simulink model "D53_LKAS_JLU_20200903_0931"  (R2018b)
settings: Solver=ode3  StartTime=0.0  StopTime=10.0  FixedStep=0.01  RelTol=1e-3  EnableMultiTasking=on
model workspace (MAT data in the model file):
  MCOS : class17 (value not decoded)
  MCOS : class17 (value not decoded)
  MCOS : class17 (value not decoded)
  MCOS : class17 (value not decoded)
  MCOS : class17 (value not decoded)
  MCOS : class17 (value not decoded)
  MCOS : class17 (value not decoded)
  MCOS : class17 (value not decoded)
  MCOS : class17 (value not decoded)
  MCOS : class17 (value not decoded)
  MCOS : class17 (value not decoded)
  MCOS : class17 (value not decoded)
  MCOS : class17 (value not decoded)
  MCOS : class17 (value not decoded)
  MCOS : class17 (value not decoded)
  MCOS : class17 (value not decoded)
  MCOS : class17 (value not decoded)
  MCOS : class17 (value not decoded)
  MCOS : class17 (value not decoded)
  MCOS : class17 (value not decoded)
  MCOS : class17 (value not decoded)
  MCOS : class17 (value not decoded)
  MCOS : class17 (value not decoded)
  MCOS : class17 (value not decoded)
  MCOS : class17 (value not decoded)
  MCOS : class17 (value not decoded)
  MCOS : class17 (value not decoded)
  MCOS : class17 (value not decoded)
  MCOS : class17 (value not decoded)
  MCOS : class17 (value not decoded)
  MCOS : class17 (value not decoded)
  MCOS : class17 (value not decoded)
  MCOS : class17 (value not decoded)
  MCOS : class17 (value not decoded)
  MCOS : class17 (value not decoded)
  MCOS : class17 (value not decoded)
  MCOS : class17 (value not decoded)
  MCOS : class17 (value not decoded)
  MCOS : class17 (value not decoded)
  MCOS : class17 (value not decoded)
  MCOS : class17 (value not decoded)
  MCOS : class17 (value not decoded)
  MCOS : class17 (value not decoded)
  MCOS : class17 (value not decoded)
  MCOS : class17 (value not decoded)
  MCOS : class17 (value not decoded)
  MCOS : class17 (value not decoded)
  MCOS : class17 (value not decoded)
  MCOS : class17 (value not decoded)
  MCOS : class17 (value not decoded)
  MCOS : class17 (value not decoded)
  MCOS : class17 (value not decoded)
  MCOS : class17 (value not decoded)
  MCOS : class17 (value not decoded)
  MCOS : class17 (value not decoded)
  MCOS : class17 (value not decoded)
  MCOS : class17 (value not decoded)
  MCOS : class17 (value not decoded)
  MCOS : class17 (value not decoded)
  MCOS : class17 (value not decoded)
  MCOS : class17 (value not decoded)
  MCOS : class17 (value not decoded)
  MCOS : class17 (value not decoded)
  MCOS : class17 (value not decoded)
  MCOS : class17 (value not decoded)
  MCOS : class17 (value not decoded)
  MCOS : class17 (value not decoded)
  MCOS : class17 (value not decoded)
  MCOS : class17 (value not decoded)
  MCOS : class17 (value not decoded)
  MCOS : class17 (value not decoded)
  MCOS : class17 (value not decoded)
  MCOS : class17 (value not decoded)
  MCOS : class17 (value not decoded)
  MCOS : class17 (value not decoded)
  MCOS : class17 (value not decoded)
  MCOS : class17 (value not decoded)
  MCOS : class17 (value not decoded)
  MCOS : class17 (value not decoded)
  MCOS : class17 (value not decoded)
  MCOS : class17 (value not decoded)
  MCOS : class17 (value not decoded)
  MCOS : class17 (value not decoded)
  MCOS : class17 (value not decoded)
  MCOS : class17 (value not decoded)
  MCOS : class17 (value not decoded)
  MCOS : class17 (value not decoded)
  MCOS : class17 (value not decoded)
  MCOS : class17 (value not decoded)
undefined symbols (not defined in the file): LKA_CarWidth, LKA_SampleTime, LKA_StrRatio_C, LKA_Veh2CamL_C, LKA_Veh2CamW_C, LKA_WhlBaseL_C, LL_CompSWA_C, LL_CrvtPrvwT_C, LL_DesDvt_C, LL_DvtComp_C, LL_DvtPrvwT_C, LL_DvtSpdDet_vDvtSpdMin_C, LL_HdAgExT_C, LL_HdAgPrvwT_C, LL_LAccMax_C, LL_LAccRMax_C, LL_LDW_EarliestWarnLine_C, LL_LDW_LatestWarnLine_C, LL_LDWS_SUPPRESS_HEADING, LL_LFClb_TFC_DiffCtlBalance, LL_LFClb_TFC_DiffCtrlMaxSWA, LL_LFClb_TFC_DiffCtrlRatio, LL_LFClb_TFC_facmGainLutGain1_C, LL_LFClb_TFC_facmGainLutGain2_C, LL_LFClb_TFC_facmIntegRatio, LL_LFClb_TFC_facmKlat_C, LL_LFClb_TFC_FfCtlRatio_C, LL_LFClb_TFC_phiIntegCtlMaxSWA_C, LL_LFClb_TFC_tiKlatPrvwT_C, LL_LFClb_TFC_vGainLutVehSpdLwr_C, LL_LFClb_TFC_vGainLutVehSpdUpr_C, LL_LKA_EarliestWarnLine_C, LL_LKA_LatestWarnLine_C, LL_LKAExPrcs_ExitC0Dvt, LL_LKAExPrcs_ExitC0Swt, LL_LKAExPrcs_tiExitTime1, LL_LKAExPrcs_tiExitTime2, LL_LKAExPrcs_tiExitTime3, LL_LKAS_OUT_OF_CONTROL_LAT_VEL, LL_LKAS_OUT_OF_CONTROL_TTLC, LL_LKASWASyn_M0, LL_LKASWASyn_M1, LL_LKASWASyn_M2, LL_LKASWASyn_M3K, LL_LKASWASyn_SWAaddMax, LL_LKASWASyn_T2, LL_LKASWASyn_tiTrqSwaRtTime, LL_LKASWASyn_tiTrqSwaTime, LL_LKASWASyn_TrqMax, LL_LKASWASyn_TrqSwaAddSwt, LL_LKASWASyn_TrqSwaRateDiff, LL_LSpdCompT_C, LL_lStpLngth_C, LL_MAX_DELAY_EPSSTAR_TIME, LL_MAX_DRIVER_TORQUE_DISABLE, LL_MAX_DRIVER_TORQUE_ENABLE, LL_MAX_LANE_WIDTH_DISABLE, LL_MAX_LANE_WIDTH_ENABLE, LL_MAX_LAT_ACC_DISABLE, LL_MAX_LAT_ACC_ENABLE ... (+30)
libraries: simulink x135, canmsglib x41, dspstat3 x3, simulink_extras x1
(part 8 of 18)

== system D53_LKAS_JLU_20200903_0931/LL/LLOn/LKA/LKA Motion Planning (LKAMP)  ==
  LKAMP_bsInInfoSyn : Inport
  LKAMP_stLKAActvFlg : Inport  Port=2
  LKAMP_bsLKAInPInfo : Inport  Port=3
  LKAMP_bsLKAClb : Inport  Port=4
  LLClb_bsConstantClb : Inport  Port=5
  Add : Sum  OutDataTypeStr=uint8
  Bus Selector : BusSelector  OutputSignals=MPInP_vVehSpdIni
  Bus Selector1 : BusSelector  OutputSignals=bsVehMovInfo.ESC_VehSpd
  Bus Selector2 : BusSelector  OutputSignals=LKA_CarWidth
  Bus Selector3 : BusSelector  OutputSignals=LL_HdAgExT_C,LL_LSpdCompT_C
  Bus Selector4 : BusSelector  OutputSignals=bsVehMovInfo.ESC_VehSpd
  Bus Selector5 : BusSelector  OutputSignals=LW_LaneWidth
  Constant : Constant  OutDataTypeStr=uint8  SampleTime=-1
  Constant19 : Constant  OutDataTypeStr=uint8  SampleTime=-1
  If : If  NumInputs=2  IfExpression=u1==u2  ShowElse=off
  LKA Motion Planning Calculation (LKAMPCal) : Subsystem  Description=|
      | Block Name: LKA Motion Planning Calculation
      | Ab.: LKAMPCal
      | No.: 1.2.3.2
      | Rev: 0.0.1
      | Update Date: 19-3-26
      settings: RTWSystemCode=Nonreusable function
  Memory1 : Memory  InheritSampleTime=on
  Motion Planning Input Processing (MPInP) : Subsystem  Description=|
      | Block Name: Motion Planning Input Processing
      | Ab.: MPInP
      | No.: 1.2.3.1
      | Rev: 0.0.1
      | Update Date: 19-3-26
  Nominal Time Calculation (NomTCalc) : Subsystem  Description=|
      | Block Name: Nominal Time Calculation
      | Ab.: NomTCalc
      | No.: 1.2.3.3
      | Rev: 0.0.1
      | Update Date: 19-3-26
  Saturation1 : Saturate  UpperLimit=5  LowerLimit=0  OutDataTypeStr=uint8
  Saturation6 : Saturate  UpperLimit=2  LowerLimit=0.2
  Steering Wheel Angle Command Calculation (SWACmdCal) : Subsystem  Description=|
      | Block Name: Steering Wheel Angle Command Calculation
      | Ab.: SWACmdCal
      | No.: 1.2.3.4
      | Rev: 0.0.1
      | Update Date: 19-3-26
  Switching Condition (SwtCon) : Subsystem
  LKAMP_phiSWACmd : Outport
  LKAMP_tiT1 : Outport  Port=2
  LKAMP_tiT2 : Outport  Port=3
  wires:
  Bus Selector5/1 -> Switching Condition (SwtCon)/4(SwtCon_lLaneWidth_C)  "<LW_LaneWidth>"
  Saturation6/1 -> LKAMP_tiT1/1
  LKAMP_bsInInfoSyn/1 -> Bus Selector4/1, Bus Selector1/1, Motion Planning Input Processing (MPInP)/4(MPInP_bsInInfoSyn)
  Bus Selector3/2 -> Switching Condition (SwtCon)/7(SwtCon_tiLSpdCompT_C)  "<LL_LSpdCompT_C>"
  LLClb_bsConstantClb/1 -> Bus Selector2/1, LKA Motion Planning Calculation (LKAMPCal)/3(LLClb_bsConstantClb)
  LKAMP_bsLKAInPInfo/1 -> Motion Planning Input Processing (MPInP)/3(MPInP_bsLKAInPInfo), Switching Condition (SwtCon)/2(SwtCon_bsLKAInPInfo), Bus Selector5/1
  Bus Selector2/1 -> Switching Condition (SwtCon)/5(SwtCon_lCarWidth_C)  "<LKA_CarWidth>"
  LKAMP_bsLKAClb/1 -> LKA Motion Planning Calculation (LKAMPCal)/2(LKAMPCal_bsLKAClb), Bus Selector3/1
  LKAMP_stLKAActvFlg/1 -> Motion Planning Input Processing (MPInP)/1(MPInP_stLKAActvFlg), Switching Condition (SwtCon)/1(SwtCon_stLKAActvFlg)
  Bus Selector4/1 -> Switching Condition (SwtCon)/3(SwtCon_vVehSpd)  "<ESC_VehSpd>"
  Bus Selector3/1 -> Switching Condition (SwtCon)/6(SwtCon_tiHdAgExTime_C)  "<LL_HdAgExT_C>"
  Saturation1/1 -> If/1, Memory1/1
  Add/1 -> Saturation1/1
  Constant19/1 -> If/2
  Constant/1 -> Add/1
  Memory1/1 -> Add/2
  If/1 -> LKA Motion Planning Calculation (LKAMPCal)/Action
  LKA Motion Planning Calculation (LKAMPCal)/1(LKAMPCal_bsLKAMPCalOut) -> Steering Wheel Angle Command Calculation (SWACmdCal)/1(SWACmdCal_bsK1K2DetOut)
  Switching Condition (SwtCon)/1(SwtCon_phiHdAgMax) -> Motion Planning Input Processing (MPInP)/2(MPInP_phiHdAgMax)
  Nominal Time Calculation (NomTCalc)/1(NomTCalc_tiNomT) -> Steering Wheel Angle Command Calculation (SWACmdCal)/3(SWACmdCal_tiNomT)
  Bus Selector1/1 -> Nominal Time Calculation (NomTCalc)/1(NomTCalc_vVehSpd)  "<ESC_VehSpd>"
  Bus Selector/1 -> Nominal Time Calculation (NomTCalc)/2(NomTCalc_vVehSpdIni)  "<MPInP_vVehSpdIni>"
  Steering Wheel Angle Command Calculation (SWACmdCal)/1(SWACmdCal_phiSWACmd) -> LKAMP_phiSWACmd/1
  Steering Wheel Angle Command Calculation (SWACmdCal)/2(SWACmdCal_tiT1) -> Saturation6/1
  Motion Planning Input Processing (MPInP)/1(MPInP_bsMPInPInfo) -> LKA Motion Planning Calculation (LKAMPCal)/1(LKAMPCal_bsLKAInPInfo), Bus Selector/1, Steering Wheel Angle Command Calculation (SWACmdCal)/2(SWACmdCal_bsLKAInPInfo)  "LKAMP_bsMPInPInfo"
  Steering Wheel Angle Command Calculation (SWACmdCal)/3(SWACmdCal_tiT2) -> LKAMP_tiT2/1

== system D53_LKAS_JLU_20200903_0931/LL/LLOn/LKA/LKA SWA Limit (LKASWALim) ==
  LKASWALim_phiTFCSWACmd : Inport
  LKASWALim_Ff : Inport  Port=2
  LKASWALim_bsLKAInPInfo : Inport  Port=3
  LKASWALim_bsLKAClb : Inport  Port=4
  Add : Sum  Inputs=+-+  OutDataTypeStr=single
  Add1 : Sum
  Add2 : Sum
  Bus Selector1 : BusSelector  OutputSignals=LKAInP_phiSWAPos,UndrLim_phiSWAMax,UndrLim_dphiSWARMax
  Bus Selector3 : BusSelector  OutputSignals=LL_CompSWA_C
  Gain1 : Gain  Gain=-1.4  OutDataTypeStr=single
  Gain2 : Gain  Gain=-1  OutDataTypeStr=single
  Gain3 : Gain  Gain=1.4  OutDataTypeStr=single
  "Rate Limiter Dynamic " : Subsystem
  Saturation Dynamic : simulink/Discontinuities/Saturation Dynamic  OutMin=[]  OutMax=[]  OutDataTypeStr=Inherit: Same as second input  OutDataType=fixdt(1, 16)  OutScaling=2^-10  DoSatur=off
  LKASWALim_phiSWACmd : Outport
  wires:
  Add2/1 -> Saturation Dynamic/3
  Add1/1 -> Saturation Dynamic/1
  LKASWALim_Ff/1 -> Add1/1, Add2/1
  Bus Selector1/1 -> Add/3  "<LKAInP_phiSWAPos>"
  LKASWALim_bsLKAInPInfo/1 -> Bus Selector1/1
  Add/1 -> Saturation Dynamic/2
  Gain1/1 -> "Rate Limiter Dynamic "/3(lo)
  Gain2/1 -> Add2/2
  Bus Selector1/3 -> Gain1/1, Gain3/1  "<UndrLim_dphiSWARMax>"
  Bus Selector1/2 -> Gain2/1, Add1/2  "<UndrLim_phiSWAMax>"
  LKASWALim_bsLKAClb/1 -> Bus Selector3/1
  LKASWALim_phiTFCSWACmd/1 -> Add/1
  Bus Selector3/1 -> Add/2  "<LL_CompSWA_C>"
  "Rate Limiter Dynamic "/1(Y) -> LKASWALim_phiSWACmd/1
  Saturation Dynamic/1 -> "Rate Limiter Dynamic "/2(u)
  Gain3/1 -> "Rate Limiter Dynamic "/1(up)

== system D53_LKAS_JLU_20200903_0931/LL/LLOn/LKA/Lane Following (LF) ==
  LF_bsInInfoSyn : Inport
  LF_bsLKAInPInfo : Inport  Port=2
  LF_bsLFClb : Inport  Port=3
  LF_bsConstantClb : Inport  Port=4
  Bus Selector4 : BusSelector  OutputSignals=LL_TFCClb
  Preview Information Calculation (PIC) : Subsystem  Description=|
      | Block Name:Preview Information Calculation
      | Ab.: PIC
      | No.: 02.01
      | Rev: 00.00.01
      | Update Date: 19-3-28
  Trajectory Following Control (TFC) : Subsystem  Description=|
      | Block Name:Trajectory Following Control
      | Ab.: TFC
      | No.: 02.02
      | Rev: 00.00.01
      | Update Date: 19-3-28
  LF_phiFfLFSWACmd : Outport
  LF_phiPropSWACmd : Outport  Port=2
  LF_phiIntegSWACmd : Outport  Port=3
  LF_phiDiffSWACmd : Outport  Port=4
  wires:
  LF_bsLKAInPInfo/1 -> Preview Information Calculation (PIC)/1(PIC_bsLKAInPInfo)
  Trajectory Following Control (TFC)/1(TFC_phiFfSWACmd) -> LF_phiFfLFSWACmd/1
  LF_bsInInfoSyn/1 -> Trajectory Following Control (TFC)/2(TFC_bsInInfoSyn)
  Preview Information Calculation (PIC)/1(PIC_bsPrvwInfo) -> Trajectory Following Control (TFC)/1(TFC_bsPrvwInfo)
  Bus Selector4/1 -> Trajectory Following Control (TFC)/3(TFC_bsTFCClb)  "<LL_TFCClb>"
  LF_bsLFClb/1 -> Bus Selector4/1
  LF_bsConstantClb/1 -> Trajectory Following Control (TFC)/4(TFC_bsConstantClb)
  Trajectory Following Control (TFC)/2(TFC_phiPropSWACmd) -> LF_phiPropSWACmd/1
  Trajectory Following Control (TFC)/3(TFC_phiIntegSWACmd) -> LF_phiIntegSWACmd/1
  Trajectory Following Control (TFC)/4(TFC_phiDiffSWACmd) -> LF_phiDiffSWACmd/1

== system D53_LKAS_JLU_20200903_0931/LL/LLOn/LKA/Plan To LaneFollowing (PTLF) ==
  InP : Inport
  Plan : Inport  Port=2
  T1 : Inport  Port=3
  DrvTrq : Inport  Port=4
  Ff : Inport  Port=5
  P : Inport  Port=6
  I : Inport  Port=7
  D : Inport  Port=8
  Add1 : Sum  Inputs=+-
  Add2 : Sum  Inputs=+-
  Add3 : Sum
  Add4 : Sum  Inputs=+++++
  Add5 : Sum  Inputs=+-
  Bus Selector1 : BusSelector  OutputSignals=Pr_bsPrInfo.bsPrCrvtInfo.crPrvwCrvt
  Bus Selector2 : BusSelector  OutputSignals=Pr_bsPrInfo.bsPrHdAgInfo.phiHdAgLft,Pr_bsPrInfo.bsPrHdAgInfo.phiHdAgRgt
  Constant1 : Constant  Value=0.1  OutDataTypeStr=single
  Constant2 : Constant  OutDataTypeStr=single
  Divide : Product  Inputs=*/
  Divide{1..2,5..7} (5 alike) : Product  Inputs=**
  Divide3 : Product  Inputs=*/
  Divide4 : Product  Inputs=*/
  InsideJudge : Subsystem
  InsideJudge1 : Subsystem
  LowPass : Subsystem
  Saturation : Saturate  UpperLimit=1  LowerLimit=0
  Saturation1 : Saturate  UpperLimit=1  LowerLimit=0
  Saturation2 : Saturate  UpperLimit=1  LowerLimit=0
  Saturation3 : Saturate  UpperLimit=0.004  LowerLimit=-0.004
  Saturation6 : Saturate  LowerLimit=0.2
  Switch : Switch  Criteria=u2 > Threshold
  TickTime (TTime) : Subsystem
      mask Display:
      | port_label('output', 1, 'TTime');
      | color('blue');
      | text(0.98,0.9,'VCDC Block','horizontalAlignment','right');
      | color('black');
      | text(0.5,0.55,'Tick Time','horizontalAlignment','center');
      | text(0.5,0.4,'(TTime)','horizontalAlignment','center');
  TimeGain : Subsystem
  SWACmd : Outport
  wires:
  InsideJudge1/2(Plan_1) -> [Plan]
  [Time] -> InsideJudge1/6(Time)
  Plan/1 -> InsideJudge1/5(Plan)
  T1/1 -> InsideJudge1/4(T1)
  Bus Selector2/2 -> InsideJudge1/3(HdAgRgt)  "<phiHdAgRgt>"
  Bus Selector2/1 -> InsideJudge1/2(HdAgLft)  "<phiHdAgLft>"
  [ActFlg] -> InsideJudge1/1(Flg)
  InP/1 -> Bus Selector1/1, Bus Selector2/1
  [Time] -> Add1/1
  Add1/1 -> Divide4/1
  [TFC] -> Divide4/2
  [T1] -> Add1/2
  [TFC] -> TimeGain/3(TFC)
  [T1] -> TimeGain/2(T1)
  [Time] -> TimeGain/1(Time)
  Saturation6/1 -> [TFC]
  InsideJudge1/1(T1_1) -> Saturation6/1, [T1]
  [T1] -> Divide3/2
  [Time] -> Add2/1
  [Time] -> Divide3/1
  Switch/1 -> Add4/4  "S_Ff"
  InsideJudge/1(Out1) -> Switch/2
  [ActFlg] -> InsideJudge/1(Flg)
  TickTime (TTime)/1(Out1) -> [Time]
  TimeGain/1(Out1) -> Divide5/1
  Divide5/1 -> Switch/1, Switch/3
  Saturation3/1 -> InsideJudge/2(Crvt)
  Bus Selector1/1 -> Saturation3/1  "<crPrvwCrvt>"
  Saturation1/1 -> Divide2/2
  [TFC] -> Divide/2
  Add4/1 -> LowPass/2(u)
  Add2/1 -> Divide/1
  [T1] -> Add2/2
  Divide3/1 -> Saturation/1
  Divide/1 -> Saturation2/1
  Saturation/1 -> Divide6/2
  Constant2/1 -> Add5/1
  Saturation2/1 -> Add5/2, Divide1/1
  [Plan] -> Divide7/1
  Divide6/1 -> Add4/5  "S_DT"
  Add5/1 -> Divide7/2
  Ff/1 -> Divide5/2
  D/1 -> Divide2/1
  DrvTrq/1 -> Divide6/1
  Divide7/1 -> Add4/1  "S_Plan"
  P/1 -> Add3/1
  I/1 -> Add3/2
  Add3/1 -> Divide1/2
  Divide1/1 -> Add4/2  "S_PI"
  Divide4/1 -> Saturation1/1
  Divide2/1 -> Add4/3  "S_D"
  LowPass/1(y) -> SWACmd/1
  [LKA_SampleTime] -> LowPass/3(dT)
  Constant1/1 -> LowPass/1(T)

== system D53_LKAS_JLU_20200903_0931/LL/LLOn/LKA Input Processing (LKAInP)/Lane Width Calculation (LW) ==
  LW_bsInInfoSyn : Inport
  Abs : Abs
  Abs1 : Abs
  Add : Sum
  Bus Selector : BusSelector  OutputSignals=bsLaneInfo.bsL0Info.L0_C0,bsLaneInfo.bsR0Info.R0_C0
  Saturation : Saturate  UpperLimit=6  LowerLimit=2
  LW_LaneWidth : Outport
  wires:
  Saturation/1 -> LW_LaneWidth/1  "LaneWidth"
  Add/1 -> Saturation/1
  Abs1/1 -> Add/2
  Abs/1 -> Add/1
  Bus Selector/2 -> Abs1/1  "<R0_C0>"
  Bus Selector/1 -> Abs/1  "<L0_C0>"
  LW_bsInInfoSyn/1 -> Bus Selector/1

== system D53_LKAS_JLU_20200903_0931/LL/LLOn/LKA Input Processing (LKAInP)/Predicted Deviation Calculation (PrDvt) ==
  PrdcDvt_stLKAActvFlg : Inport
  PrdcDvt_bsInInfoSyn : Inport  Port=2
  PrdcDvt_bsPrdcHdAgInfo : Inport  Port=3
  PrdcDvt_bsLKAClb : Inport  Port=4
  Bus Creator1 : BusCreator  Inputs=8
  Bus Selector : BusSelector  OutputSignals=bsLaneInfo.bsL0Info,bsVehMovInfo.ESC_VehSpd,bsLaneInfo.bsR0Info
  Bus Selector1 : BusSelector  OutputSignals=LL_DvtPrvwT_C,LL_DvtComp_C
  Bus Selector2 : BusSelector  OutputSignals=bsLaneInfo.bsL0Info.L0_C0,bsLaneInfo.bsR0Info.R0_C0
  Bus Selector3 : BusSelector  OutputSignals=EnaCClb.LL_DvtComp_C
  Lane Information Selection (LaneInfoSel) : Subsystem
  Lane Information Selection (LaneInfoSel)1 : Subsystem
  Left Front Conner Deviation Calculation (LFCDvtCalc) : Subsystem
  Predicted Deviation Correction (PrdcDvtCor) : Subsystem
  Predicted Deviation of Left Lane Line (PrdcDvtLft) : Subsystem
  Predicted Deviation of Left Line (PrdcDvtLft) : Subsystem
  Predicted Deviation of Right  Line (PrdcDvtRgt) : Subsystem
  Predicted Deviation of Right Lane Line (PrdcDvtRgt) : Subsystem
  Right Front Conner Deviation Calculation (RFCDvtCalc) : Subsystem
  Z Calculation (ZCalc) : Subsystem
  PrdcDvt_bsPrdcDvtInfo : Outport
  wires:
  Lane Information Selection (LaneInfoSel)1/1(LaneInfoSel_facmActvLane) -> Bus Creator1/6  "lDvt"
  Right Front Conner Deviation Calculation (RFCDvtCalc)/1(DvtCalc_lRgtDvt) -> Bus Creator1/8, Lane Information Selection (LaneInfoSel)1/3(LaneInfoSel_facmRgtLane)  "IRgtDvt"
  Left Front Conner Deviation Calculation (LFCDvtCalc)/1(DvtCalc_lLftDvt) -> Bus Creator1/7, Lane Information Selection (LaneInfoSel)1/2(LaneInfoSel_facmLftLane)  "ILftDvt"
  Bus Selector3/1 -> Left Front Conner Deviation Calculation (LFCDvtCalc)/3(LFCDvtCalc_lDvtComp_C), Right Front Conner Deviation Calculation (RFCDvtCalc)/1(RFCDvtCalc_lDvtComp_C)  "<LL_DvtComp_C>"
  [LLClb_bsLLSMConClb] -> Bus Selector3/1
  Bus Selector2/2 -> Right Front Conner Deviation Calculation (RFCDvtCalc)/2(RFCDvtCalc_lDvt)  "<R0_C0>"
  Bus Selector2/1 -> Left Front Conner Deviation Calculation (LFCDvtCalc)/2(LFCDvtCalc_lDvt)  "<L0_C0>"
  Lane Information Selection (LaneInfoSel)/1(LaneInfoSel_facmActvLane) -> Bus Creator1/1  "lPrdcDvt"
  PrdcDvt_stLKAActvFlg/1 -> Lane Information Selection (LaneInfoSel)1/1(LaneInfoSel_stLKAActvFlg), Lane Information Selection (LaneInfoSel)/1(LaneInfoSel_stLKAActvFlg)
  Bus Creator1/1 -> PrdcDvt_bsPrdcDvtInfo/1
  Predicted Deviation of Right  Line (PrdcDvtRgt)/1(PrdcDvtLft_lDvtRgt) -> Bus Creator1/3, Lane Information Selection (LaneInfoSel)/3(LaneInfoSel_facmRgtLane)  "lPrdcDvtRgt"
  Predicted Deviation of Left Line (PrdcDvtLft)/1(PrdcDvtLft_lDvtLft) -> Lane Information Selection (LaneInfoSel)/2(LaneInfoSel_facmLftLane), Bus Creator1/2  "lPrdcDvtLft"
  Predicted Deviation of Left Lane Line (PrdcDvtLft)/1(PrdcDvtLft_lPrdcDvtLft) -> Predicted Deviation of Left Line (PrdcDvtLft)/3(PrdcDvtLft_lPrdcDvtLft), Bus Creator1/4  "lPrvwDvtLft"
  Bus Selector/3 -> Predicted Deviation of Right Lane Line (PrdcDvtRgt)/2(PrdcDvtRgt_bsR0Info)  "<bsR0Info>"
  Bus Selector/2 -> Z Calculation (ZCalc)/1(ZCalc_vVehSpd)  "<ESC_VehSpd>"
  Predicted Deviation of Right Lane Line (PrdcDvtRgt)/1(PrdcDvtRgt_lPrdcDvtRgt) -> Predicted Deviation of Right  Line (PrdcDvtRgt)/3(PrdcDvtLft_lPrdcDvtLft), Bus Creator1/5  "lPrvwDvtRgt"
  Z Calculation (ZCalc)/1(ZCalc_lPrvwDstZ) -> Predicted Deviation Correction (PrdcDvtCor)/2(PrdcDvtCor_lPrvwDstZ), Predicted Deviation of Left Lane Line (PrdcDvtLft)/2(PrdcDvtLft_lPrvwDstZ), Predicted Deviation of Right Lane Line (PrdcDvtRgt)/1(PrdcDvtRgt_lPrvwDstZ)
  PrdcDvt_bsInInfoSyn/1 -> Bus Selector/1, Bus Selector2/1
  Bus Selector/1 -> Predicted Deviation of Left Lane Line (PrdcDvtLft)/1(PrdcDvtLft_bsL0Info)  "<bsL0Info>"
  PrdcDvt_bsPrdcHdAgInfo/1 -> Predicted Deviation of Left Line (PrdcDvtLft)/1(PrdcDvtLft_bsPrdcHdAgInfo), Predicted Deviation of Right  Line (PrdcDvtRgt)/1(PrdcDvtLft_bsPrdcHdAgInfo), Predicted Deviation Correction (PrdcDvtCor)/1(PrdcDvtCor_bsPrdcHdAgInfo), Left Front Conner Deviation Calculation (LFCDvtCalc)/1(PrdcDvt_bsPrHdAgInfo), Right Front Conner Deviation Calculation (RFCDvtCalc)/3(PrdcDvt_bsPrHdAgInfo)
  Predicted Deviation Correction (PrdcDvtCor)/1(PrdcDvtCor_lPrdcDvtCor) -> Predicted Deviation of Left Line (PrdcDvtLft)/2(PrdcDvtLft_lPrdcDvtCor), Predicted Deviation of Right  Line (PrdcDvtRgt)/2(PrdcDvtLft_lPrdcDvtCor)
  PrdcDvt_bsLKAClb/1 -> Bus Selector1/1
  Bus Selector1/1 -> Z Calculation (ZCalc)/2(ZCalc_tiDvtPrvwT_C)  "<LL_DvtPrvwT_C>"
  Bus Selector1/2 -> Predicted Deviation of Right  Line (PrdcDvtRgt)/4(PrdcDvtLft_lDvtComp_C), Predicted Deviation of Left Line (PrdcDvtLft)/4(PrdcDvtLft_lDvtComp_C)  "<LL_DvtComp_C>"

== system D53_LKAS_JLU_20200903_0931/LL/LLOn/LKA Input Processing (LKAInP)/Predicted Heading Angle Calculation (PrHdAg) ==
  PrHdAg_bsTTLCInfo : Inport
  PrdcHdAg_stLKAActvFlg : Inport  Port=2
  PrHdAg_bsInInfoSyn : Inport  Port=3
  PrHdAg_bsLKAClb : Inport  Port=4
  Add : Sum  OutDataTypeStr=single
  Add1 : Sum  OutDataTypeStr=single
  Bus Creator : BusCreator  Inputs=10
  Bus Selector : BusSelector  OutputSignals=bsLaneInfo.bsL0Info,bsVehMovInfo.ESC_VehSpd,bsLaneInfo.bsR0Info,bsSWAInfo.SW_Angle
  Bus Selector1 : BusSelector  OutputSignals=LL_HdAgPrvwT_C
  Bus Selector2 : BusSelector  OutputSignals=LFTTTLC,RGTTTLC
  Heading Angle (HdAg) : Subsystem
  Lane Information Selection (LaneInfoSel) : Subsystem
  Lane Information Selection (LaneInfoSel)1 : Subsystem
  Min : MinMax  Inputs=2
  Perdicted Heading Angle Compensation (PrdcHdAgComp) : Subsystem
  Perdicted Heading Angle from Right Lane Line (PrdcHdAgRgt) : Subsystem
  Perdicted Heading Angle from Right Lane Line (PrdcHdAgRgt)1 : Subsystem
  Predicted Heading Angle from Left Lane Line (PrdcHdAgtLft) : Subsystem
  Predicted Heading Angle from Left Lane Line (PrdcHdAgtLft)1 : Subsystem
  Saturation : Saturate  UpperLimit=2  LowerLimit=0.5
  Z Calculation (ZCalc) : Subsystem
  Z Calculation (ZCalc)1 : Subsystem
  PrHdAg_bsPrHdAgInfo : Outport
  wires:
  Perdicted Heading Angle from Right Lane Line (PrdcHdAgRgt)1/1(PrdcHdAgRgt_phiPrdcHdAgRgt) -> Bus Creator/10  "phiPrvwHdAgRgt"
  Predicted Heading Angle from Left Lane Line (PrdcHdAgtLft)1/1(PrdcHdAgtLft_phiPrdcHdAgLft) -> Bus Creator/9  "phiPrvwHdAgLft"
  Z Calculation (ZCalc)1/1(ZCalc_lPrvwDstZ) -> Predicted Heading Angle from Left Lane Line (PrdcHdAgtLft)1/2(PrdcHdAgtLft_lPrvwDstZ), Perdicted Heading Angle from Right Lane Line (PrdcHdAgRgt)1/1(PrdcHdAgRgt_lPrvwDstZ)
  Bus Selector1/1 -> Z Calculation (ZCalc)1/2(ZCalc_tiHdAgPrvwT_C)  "<LL_HdAgPrvwT_C>"
  PrHdAg_bsLKAClb/1 -> Bus Selector1/1
  Heading Angle (HdAg)/3(HdAg_phiHdAgRgt) -> Bus Creator/8  "phiHdAgRgt"
  Heading Angle (HdAg)/2(HdAg_phiHdAgLft) -> Bus Creator/7  "phiHdAgLft"
  Heading Angle (HdAg)/1(HdAg_phiHdAg) -> Bus Creator/6  "phiHdAg"
  Saturation/1 -> Perdicted Heading Angle Compensation (PrdcHdAgComp)/3(PrdcHdAgComp_tiHdAgPrvwT_C), Z Calculation (ZCalc)/2(ZCalc_tiHdAgPrvwT_C)
  Bus Selector2/2 -> Min/2  "<RGTTTLC>"
  Bus Selector2/1 -> Min/1  "<LFTTTLC>"
  PrHdAg_bsTTLCInfo/1 -> Bus Selector2/1
  Lane Information Selection (LaneInfoSel)1/1(LaneInfoSel_facmActvLane) -> Bus Creator/2  "phiPrvwTTLCHdAg"
  Bus Selector/1 -> Predicted Heading Angle from Left Lane Line (PrdcHdAgtLft)/1(PrdcHdAgtLft_bsL0Info), Predicted Heading Angle from Left Lane Line (PrdcHdAgtLft)1/1(PrdcHdAgtLft_bsL0Info)  "<bsL0Info>"
  Z Calculation (ZCalc)/1(ZCalc_lPrvwDstZ) -> Predicted Heading Angle from Left Lane Line (PrdcHdAgtLft)/2(PrdcHdAgtLft_lPrvwDstZ), Perdicted Heading Angle from Right Lane Line (PrdcHdAgRgt)/1(PrdcHdAgRgt_lPrvwDstZ)
  Lane Information Selection (LaneInfoSel)/1(LaneInfoSel_facmActvLane) -> Bus Creator/1  "phiPrdcTTLCHdAg"
  PrdcHdAg_stLKAActvFlg/1 -> Lane Information Selection (LaneInfoSel)/1(LaneInfoSel_stLKAActvFlg), Lane Information Selection (LaneInfoSel)1/1(LaneInfoSel_stLKAActvFlg)
  Add1/1 -> Lane Information Selection (LaneInfoSel)/3(LaneInfoSel_facmRgtLane)  "phiPrdcHdAgRgt"
  Add/1 -> Lane Information Selection (LaneInfoSel)/2(LaneInfoSel_facmLftLane)  "phiPrdcHdAgLft"
  Perdicted Heading Angle Compensation (PrdcHdAgComp)/1(PrdcHdAgComp_phiPrdcHdAgComp) -> Add1/2, Bus Creator/5, Add/2  "phiPrdcHdAgComp"
  Predicted Heading Angle from Left Lane Line (PrdcHdAgtLft)/1(PrdcHdAgtLft_phiPrdcHdAgLft) -> Add/1, Bus Creator/3, Lane Information Selection (LaneInfoSel)1/2(LaneInfoSel_facmLftLane)  "phiPrvwTTLCHdAgLft"
  Perdicted Heading Angle from Right Lane Line (PrdcHdAgRgt)/1(PrdcHdAgRgt_phiPrdcHdAgRgt) -> Add1/1, Lane Information Selection (LaneInfoSel)1/3(LaneInfoSel_facmRgtLane), Bus Creator/4  "phiPrvwTTLCHdAgRgt"
  Bus Creator/1 -> PrHdAg_bsPrHdAgInfo/1
  PrHdAg_bsInInfoSyn/1 -> Bus Selector/1, Heading Angle (HdAg)/1(HdAg_bsLaneInfo)
  Bus Selector/2 -> Z Calculation (ZCalc)/1(ZCalc_vVehSpd), Perdicted Heading Angle Compensation (PrdcHdAgComp)/1(PrdcHdAgComp_vVehSpd), Z Calculation (ZCalc)1/1(ZCalc_vVehSpd)  "<ESC_VehSpd>"
  Bus Selector/3 -> Perdicted Heading Angle from Right Lane Line (PrdcHdAgRgt)/2(PrdcHdAgRgt_bsR0Info), Perdicted Heading Angle from Right Lane Line (PrdcHdAgRgt)1/2(PrdcHdAgRgt_bsR0Info)  "<bsR0Info>"
  Bus Selector/4 -> Perdicted Heading Angle Compensation (PrdcHdAgComp)/2(PrdcHdAgComp_phiSWA)  "<SW_Angle>"
  Min/1 -> Saturation/1

== system D53_LKAS_JLU_20200903_0931/LL/LLOn/LKA Input Processing (LKAInP)/Previewed Curvature (PrCrvt) ==
  PrvwCrvt_stLKAActvFlg : Inport
  PrvwCrvt_bsInInfoSyn : Inport  Port=2
  PrvwCrvt_tiCrvtPrvwT_C : Inport  Port=3
  Bus Creator : BusCreator  Inputs=3
  Bus Selector : BusSelector  OutputSignals=LL_CrvtPrvwT_C
  Bus Selector2 : BusSelector  OutputSignals=bsLaneInfo.bsL0Info,bsVehMovInfo.ESC_VehSpd,bsLaneInfo.bsR0Info
  Curvature Ahead of Left Lane Line (CrvtAhdLft) : Subsystem
  Curvature Ahead of Left Lane Line (CrvtAhdLft)1 : Subsystem
  Lane Information Selection (LaneInfoSel) : Subsystem
  Z Calculation (ZCalc) : Subsystem
  PrvwCrvt_bsPrvwCrvtInfo : Outport
  wires:
  Bus Creator/1 -> PrvwCrvt_bsPrvwCrvtInfo/1
  Lane Information Selection (LaneInfoSel)/1(LaneInfoSel_facmActvLane) -> Bus Creator/1  "crPrvwCrvt"
  Curvature Ahead of Left Lane Line (CrvtAhdLft)1/1(CrvtAhdRgt_crCrvtAhdRgt) -> Bus Creator/3, Lane Information Selection (LaneInfoSel)/3(LaneInfoSel_facmRgtLane)  "crPrvwCrvtRgt"
  Curvature Ahead of Left Lane Line (CrvtAhdLft)/1(CrvtAhdLft_crCrvtAhdLft) -> Lane Information Selection (LaneInfoSel)/2(LaneInfoSel_facmLftLane), Bus Creator/2  "crPrvwCrvtLft"
  PrvwCrvt_stLKAActvFlg/1 -> Lane Information Selection (LaneInfoSel)/1(LaneInfoSel_stLKAActvFlg)
  Bus Selector/1 -> Z Calculation (ZCalc)/2(ZCalc_tiCrvtPrvwT_C)  "<LL_CrvtPrvwT_C>"
  PrvwCrvt_tiCrvtPrvwT_C/1 -> Bus Selector/1
  Bus Selector2/2 -> Z Calculation (ZCalc)/1(ZCalc_vVehSpd)  "<ESC_VehSpd>"
  Bus Selector2/3 -> Curvature Ahead of Left Lane Line (CrvtAhdLft)1/2(CrvtAhdRgt_bsR0Info)  "<bsR0Info>"
  Bus Selector2/1 -> Curvature Ahead of Left Lane Line (CrvtAhdLft)/1(CrvtAhdLft_bsL0Info)  "<bsL0Info>"
  Z Calculation (ZCalc)/1(ZCalc_lPrvwDstZ) -> Curvature Ahead of Left Lane Line (CrvtAhdLft)/2(CrvtAhdLft_lPrvwDstZ), Curvature Ahead of Left Lane Line (CrvtAhdLft)1/1(CrvtAhdRgt_lPrvwDstZ)
  PrvwCrvt_bsInInfoSyn/1 -> Bus Selector2/1

== system D53_LKAS_JLU_20200903_0931/LL/LLOn/LKA Input Processing (LKAInP)/Steering Wheel Position Calculation (SWAPosCal) ==
  SWAPosCal_bsInInfoSyn : Inport
  Bus Selector : BusSelector  OutputSignals=bsLaneInfo.bsL0Info,bsLaneInfo.bsR0Info,bsVehMovInfo.ESC_VehSpd,bsSWAInfo.SW_Angle
  Bus Selector2 : BusSelector  OutputSignals=LKA_SampleTime
  Subsystem : Subsystem
  Subsystem1 : Subsystem
  SWAPosCal : Outport
  wires:
  Bus Selector2/1 -> Subsystem/2(<LKA_SampleTime>)  "<LKA_SampleTime>"
  [LLClb_bsConstantClb] -> Bus Selector2/1
  Subsystem/1(SWAPos) -> SWAPosCal/1
  Bus Selector/4 -> Subsystem1/4(SWA), Subsystem/1(SWAIn)  "<SW_Angle>"
  Bus Selector/3 -> Subsystem1/3(VehSpd)  "<ESC_VehSpd>"
  Subsystem1/1(Flg) -> Subsystem/Enable  "SWAPosEna"
  Bus Selector/2 -> Subsystem1/2(R0)  "<bsR0Info>"
  Bus Selector/1 -> Subsystem1/1(L0)  "<bsL0Info>"
  SWAPosCal_bsInInfoSyn/1 -> Bus Selector/1

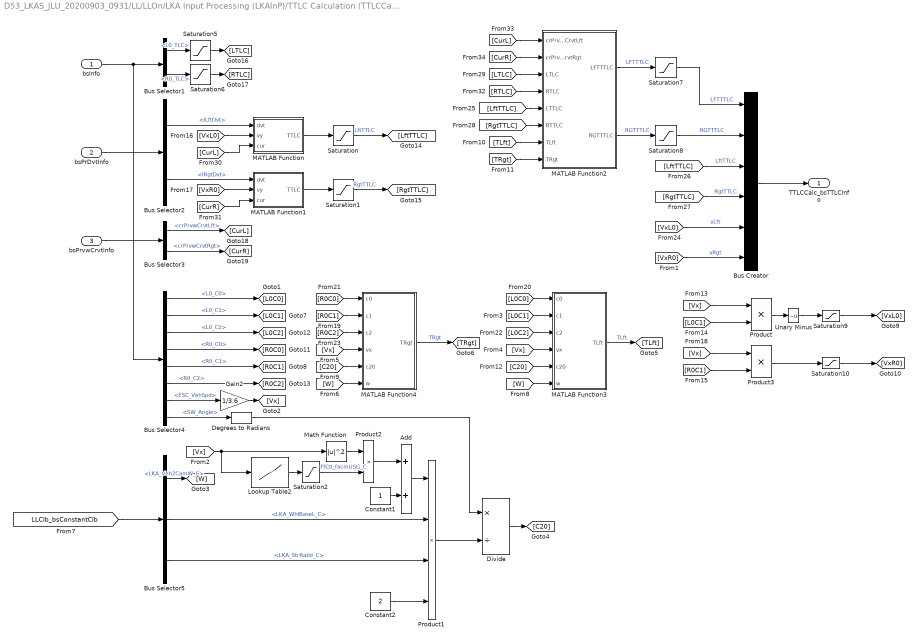
== system D53_LKAS_JLU_20200903_0931/LL/LLOn/LKA Input Processing (LKAInP)/TTLC Calculation (TTLCCalc) ==
  bsInfo : Inport
  bsPrDvtInfo : Inport  Port=2
  bsPrvwCrvtInfo : Inport  Port=3
  Add : Sum  OutDataTypeStr=single
  Bus Creator : BusCreator  Inputs=6
  Bus Selector1 : BusSelector  OutputSignals=bsLaneInfo.bsL0Info.L0_TLC,bsLaneInfo.bsR0Info.R0_TLC
  Bus Selector2 : BusSelector  OutputSignals=ILftDvt,IRgtDvt
  Bus Selector3 : BusSelector  OutputSignals=crPrvwCrvtLft,crPrvwCrvtRgt
  Bus Selector4 : BusSelector  OutputSignals=bsLaneInfo.bsL0Info.L0_C0,bsLaneInfo.bsL0Info.L0_C1,bsLaneInfo.bsL0Info.L0_C2,bsLaneInfo.bsR0Info.R0_C0,bsLaneInfo.bsR0Info.R0_C1,bsLaneInfo.bsR0Info.R0_C2,bsVehMovInfo.ESC_VehSpd,bsSWAInfo.SW_Angle
  Bus Selector5 : BusSelector  OutputSignals=LKA_Veh2CamW_C,LKA_WhlBaseL_C,LKA_StrRatio_C
  Constant1 : Constant  OutDataTypeStr=single
  Constant2 : Constant  Value=2  OutDataTypeStr=single
  Degrees to Radians : simulink_extras/Transformations/Degrees to Radians
  Divide : Product  Inputs=*/
  Gain2 : Gain  Gain=1/3.6
  Lookup Table2 : Lookup_n-D  NumberOfTableDimensions=1  BreakpointsForDimension1=[11.7,18.83,26.98,31.98,51.04,79,86.08,90.59]  BeginIndexSearchUsingPreviousIndexResult=on  Table=[0.012141,0.005179,0.00298,0.002547,0.001715,0.001283,0.001021,0.000982]  DiagnosticForOutOfRangeInput=Warning  RemoveProtectionInput=on  InternalRulePriority=Speed  OutDataTypeStr=single  RndMeth=Simplest  InputSameDT=on
  MATLAB Function : MATLAB Function  TreatAsAtomicUnit=on
  MATLAB Function1 : MATLAB Function  TreatAsAtomicUnit=on
  MATLAB Function2 : MATLAB Function  TreatAsAtomicUnit=on
  MATLAB Function3 : MATLAB Function  TreatAsAtomicUnit=on
  MATLAB Function4 : MATLAB Function  TreatAsAtomicUnit=on
  Math Function : Math  Operator=magnitude^2  OutDataTypeStr=single  SaturateOnIntegerOverflow=on
  Product : Product
  Product1 : Product  Inputs=4  OutDataTypeStr=single
  Product2 : Product  OutDataTypeStr=single
  Product3 : Product
  Saturation : Saturate  UpperLimit=2  LowerLimit=0.6  OutDataTypeStr=single
  Saturation1 : Saturate  UpperLimit=2  LowerLimit=0.6  OutDataTypeStr=single
  Saturation10 : Saturate  UpperLimit=1  LowerLimit=-1
  Saturation2 : Saturate  UpperLimit=0.01  LowerLimit=0
  Saturation5 : Saturate  UpperLimit=2  LowerLimit=0.6
  Saturation6 : Saturate  UpperLimit=2  LowerLimit=0.6
  Saturation7 : Saturate  UpperLimit=2  LowerLimit=0.8
  Saturation8 : Saturate  UpperLimit=2  LowerLimit=0.8
  Saturation9 : Saturate  UpperLimit=1  LowerLimit=-1
  Unary Minus : UnaryMinus
  TTLCCalc_bsTTLCInfo : Outport
  wires:
  Constant2/1 -> Product1/4
  [CurR] -> MATLAB Function2/2(crPrvwCrvtRgt)
  Saturation8/1 -> Bus Creator/2  "RGTTTLC"
  MATLAB Function2/2(RGTTTLC) -> Saturation8/1  "RGTTTLC"
  [LTLC] -> MATLAB Function2/3(LTLC)
  [RgtTTLC] -> MATLAB Function2/6(RTTLC)
  [RgtTTLC] -> Bus Creator/4  "RgtTTLC"
  [RTLC] -> MATLAB Function2/4(RTLC)
  MATLAB Function2/1(LFTTTLC) -> Saturation7/1  "LFTTTLC"
  [CurL] -> MATLAB Function2/1(crPrvwCrvtLft)
  Saturation7/1 -> Bus Creator/1  "LFTTTLC"
  [LftTTLC] -> Bus Creator/3  "LftTTLC"
  [TRgt] -> MATLAB Function2/8(TRgt)
  [LftTTLC] -> MATLAB Function2/5(LTTLC)
  [TLft] -> MATLAB Function2/7(TLft)
  Bus Creator/1 -> TTLCCalc_bsTTLCInfo/1
  [VxL0] -> Bus Creator/5  "vLft"
  [VxR0] -> Bus Creator/6  "vRgt"
  Saturation10/1 -> [VxR0]
  Unary Minus/1 -> Saturation9/1
  [R0C1] -> Product3/2
  Product/1 -> Unary Minus/1
  Saturation9/1 -> [VxL0]
  [Vx] -> Product/1
  [L0C1] -> Product/2
  [Vx] -> Product3/1
  Product3/1 -> Saturation10/1
  [L0C0] -> MATLAB Function3/1(c0)
  [L0C2] -> MATLAB Function3/3(c2)
  [Vx] -> MATLAB Function4/4(vx)
  [R0C1] -> MATLAB Function4/2(c1)
  [W] -> MATLAB Function3/6(w)
  [L0C1] -> MATLAB Function3/2(c1)
  MATLAB Function3/1(TLft) -> [TLft]  "TLft"
  [R0C0] -> MATLAB Function4/1(c0)
  [W] -> MATLAB Function4/6(w)
  [C20] -> MATLAB Function4/5(c20)
  [Vx] -> MATLAB Function3/4(vx)
  [R0C2] -> MATLAB Function4/3(c2)
  MATLAB Function4/1(TRgt) -> [TRgt]  "TRgt"
  [C20] -> MATLAB Function3/5(c20)
  Bus Selector4/3 -> [L0C2]  "<L0_C2>"
  Bus Selector4/1 -> [L0C0]  "<L0_C0>"
  Bus Selector4/2 -> [L0C1]  "<L0_C1>"
  Bus Selector4/6 -> [R0C2]  "<R0_C2>"
  Bus Selector4/4 -> [R0C0]  "<R0_C0>"
  Bus Selector4/5 -> [R0C1]  "<R0_C1>"
  Bus Selector3/2 -> [CurR]  "<crPrvwCrvtRgt>"
  Bus Selector3/1 -> [CurL]  "<crPrvwCrvtLft>"
  [CurL] -> MATLAB Function/3(cur)
  [CurR] -> MATLAB Function1/3(cur)
  Bus Selector2/1 -> MATLAB Function/1(dvt)  "<ILftDvt>"
  Saturation1/1 -> [RgtTTLC]  "RgtTTLC"
  Saturation/1 -> [LftTTLC]  "LftTTLC"
  MATLAB Function/1(TTLC) -> Saturation/1
  MATLAB Function1/1(TTLC) -> Saturation1/1
  [VxR0] -> MATLAB Function1/2(vy)
  [VxL0] -> MATLAB Function/2(vy)
  Bus Selector2/2 -> MATLAB Function1/1(dvt)  "<IRgtDvt>"
  Bus Selector1/2 -> Saturation6/1  "<R0_TLC>"
  Bus Selector1/1 -> Saturation5/1  "<L0_TLC>"
  Saturation5/1 -> [LTLC]
  Saturation6/1 -> [RTLC]
  bsPrvwCrvtInfo/1 -> Bus Selector3/1
  bsPrDvtInfo/1 -> Bus Selector2/1
  bsInfo/1 -> Bus Selector4/1, Bus Selector1/1
  [LLClb_bsConstantClb] -> Bus Selector5/1
  Product2/1 -> Add/1
  Math Function/1 -> Product2/1
  Lookup Table2/1 -> Saturation2/1
  Constant1/1 -> Add/2
  Saturation2/1 -> Product2/2  "FfCtl_facmUSG_C"
  Bus Selector4/7 -> Gain2/1  "<ESC_VehSpd>"
  Add/1 -> Product1/1
  Bus Selector5/2 -> Product1/2  "<LKA_WhlBaseL_C>"
  Bus Selector5/3 -> Product1/3  "<LKA_StrRatio_C>"
  Product1/1 -> Divide/2
  Bus Selector4/8 -> Degrees to Radians/1  "<SW_Angle>"
  Degrees to Radians/1 -> Divide/1
  Gain2/1 -> [Vx]
  [Vx] -> Lookup Table2/1, Math Function/1
  Bus Selector5/1 -> [W]  "<LKA_Veh2CamW_C>"
  Divide/1 -> [C20]

== system D53_LKAS_JLU_20200903_0931/LL/LLOn/LKA Input Processing (LKAInP)/Under The Limit (UndrLim) ==
  UndrLim_bsInInfoSyn : Inport
  UndrLim_bsUndrLimClb : Inport  Port=2
  Bus Selector : BusSelector  OutputSignals=LL_LAccMax_C,LL_LAccRMax_C
  Bus Selector1 : BusSelector  OutputSignals=bsVehMovInfo.ESC_VehSpd
  Bus Selector2 : BusSelector  OutputSignals=LKA_StrRatio_C,LKA_WhlBaseL_C
  Saturation : Saturate  UpperLimit=150  LowerLimit=0.001
  Steering Wheel Angel Max (SWAMax) : Subsystem
  Steering Wheel Angel Rate Max (SWARMax) : Subsystem
  UndrLim_phiSWAMax : Outport
  UndrLim_dphiSWARMax : Outport  Port=2
  wires:
  [LLClb_bsConstantClb] -> Bus Selector2/1
  Bus Selector2/2 -> Steering Wheel Angel Rate Max (SWARMax)/4(LKA_WhlBaseL_C), Steering Wheel Angel Max (SWAMax)/4(LKA_WhlBaseL_C)  "<LKA_WhlBaseL_C>"
  Bus Selector2/1 -> Steering Wheel Angel Rate Max (SWARMax)/3(LKA_StrRatio_C), Steering Wheel Angel Max (SWAMax)/3(LKA_StrRatio_C)  "<LKA_StrRatio_C>"
  Bus Selector1/1 -> Saturation/1  "<ESC_VehSpd>"
  UndrLim_bsInInfoSyn/1 -> Bus Selector1/1
  Bus Selector/2 -> Steering Wheel Angel Rate Max (SWARMax)/2(SWARateMax_aLAccR_C)  "<LL_LAccRMax_C>"
  Bus Selector/1 -> Steering Wheel Angel Max (SWAMax)/2(SWAMax_aLAcc_C)  "<LL_LAccMax_C>"
  UndrLim_bsUndrLimClb/1 -> Bus Selector/1
  Steering Wheel Angel Max (SWAMax)/1(SWAMax_phiSWAMax) -> UndrLim_phiSWAMax/1
  Steering Wheel Angel Rate Max (SWARMax)/1(SWARMax_dphiSWARMax) -> UndrLim_dphiSWARMax/1
  Saturation/1 -> Steering Wheel Angel Max (SWAMax)/1(SWAMax_vVehSpd), Steering Wheel Angel Rate Max (SWARMax)/1(SWARateMax_vVehSpd)

== system D53_LKAS_JLU_20200903_0931/LL/LLOn/LL State Determination (LLStateDet)/LL State Machine Conditions (LLSMCon) ==
  LLSMCon_stDACModeIn : Inport
  LLSMCon_bsInInfoSyn : Inport  Port=2
  LLSMCon_bsLKAInPInfo : Inport  Port=3
  LLSMCon_bsLLSMConClb : Inport  Port=4
  LLSMCon_bsLLState : Inport  Port=5
  LLSMCon_stExitFlg : Inport  Port=6
  LLSMCon_bsSignalFault : Inport  Port=7
  Activation Condition (ActvC) : Subsystem  Description=|
      | Block Name: Activation Condition
      | Ab.: ActvC
      | No.: 1.1.1.4.0.
      | Rev: 0.0.1
      | Update Date: 19-3-26
  Deactivation Condition (DeactvC) : Subsystem  Description=|
      | Block Name: Deactivation Condition
      | Ab.: DeactvC
      | No.: 1.1.1.5.0.0
      | Rev: 0.0.1
      | Update Date: 19-3-26
  Disable Condition (DisblC) : Subsystem  Description=|
      | Block Name: Disable Condition
      | Ab.: DisblC
      | No.: 1.1.1.3.0.0
      | Rev: 0.0.1
      | Update Date: 19-3-26
  Enable Condition (EnaC) : Subsystem  Description=|
      | Block Name: Enable Condition
      | Ab.: EnaC
      | No.: 1.1.1.2.0.0
      | Rev: 0.0.1
      | Update Date: 19-3-26
      settings: PermitHierarchicalResolution=None  MinAlgLoopOccurrences=on
  Fault Condition (FaultC) : Subsystem  Description=|
      | Block Name: Fault Condition
      | Ab.: FaultC
      | No.: 1.1.1.6.0.0
      | Rev: 0.0.1
      | Update Date: 19-3-26
  LLSMCon_stDACMode : Outport
  LLSMCon_stLDWEnaCSyn : Outport  Port=2
  LLSMCon_stLDWDisblCSyn : Outport  Port=3
  LLSMCon_stLDWActvCSyn : Outport  Port=4
  LLSMCon_stLDWDeactvCSyn : Outport  Port=5
  LLSMCon_stLDWFaultCSyn : Outport  Port=6
  LLSMCon_stLKAEnaCSyn : Outport  Port=7
  LLSMCon_stLKADisblCSyn : Outport  Port=8
  LLSMCon_stLKAActvCSyn : Outport  Port=9
  LLSMCon_stLKADeactvCSyn : Outport  Port=10
  LLSMCon_stLKAFaultCSyn : Outport  Port=11
  wires:
  LLSMCon_bsLKAInPInfo/1 -> Enable Condition (EnaC)/3(EnaC_bsLKAInPInfo), Disable Condition (DisblC)/3(LKAInPInfo), Activation Condition (ActvC)/3(LKAInPInfo), Deactivation Condition (DeactvC)/3(LKAInPInfo)
  LLSMCon_bsSignalFault/1 -> Fault Condition (FaultC)/2(FaultC_SignalFault)
  Activation Condition (ActvC)/2(ActvC_stLKAActvCSyn) -> LLSMCon_stLKAActvCSyn/1
  LLSMCon_bsLLSMConClb/1 -> Enable Condition (EnaC)/4(EnaC_bsLLSMConClb), Disable Condition (DisblC)/4(LLSMConClb), Activation Condition (ActvC)/4(LLSMConClb), Deactivation Condition (DeactvC)/4(LLSMConClb)
  LLSMCon_stExitFlg/1 -> Deactivation Condition (DeactvC)/6(ExitFlg)
  Deactivation Condition (DeactvC)/1(DeactvC_stLDWDeactvCSyn) -> LLSMCon_stLDWDeactvCSyn/1
  Fault Condition (FaultC)/2(FaultC_stLKAFaultCSyn) -> LLSMCon_stLKAFaultCSyn/1
  Deactivation Condition (DeactvC)/2(DeactvC_stLKADeactvCSyn) -> LLSMCon_stLKADeactvCSyn/1
  Fault Condition (FaultC)/1(FaultC_stLDWFaultCSyn) -> LLSMCon_stLDWFaultCSyn/1
  LLSMCon_stDACModeIn/1 -> Enable Condition (EnaC)/1(EnaC_stDACMode), Disable Condition (DisblC)/1(DACMode), Activation Condition (ActvC)/1(DACMode), Deactivation Condition (DeactvC)/1(DACMode), LLSMCon_stDACMode/1
  Activation Condition (ActvC)/1(ActvC_stLDWActvCSyn) -> LLSMCon_stLDWActvCSyn/1
  LLSMCon_bsInInfoSyn/1 -> Disable Condition (DisblC)/2(InInfoSyn), Activation Condition (ActvC)/2(InInfoSyn), Deactivation Condition (DeactvC)/2(InInfoSyn), Fault Condition (FaultC)/1(FaultC_bsInInfoSyn), Enable Condition (EnaC)/2(EnaC_bsInInfoSyn)
  LLSMCon_bsLLState/1 -> Disable Condition (DisblC)/5(LLState), Deactivation Condition (DeactvC)/5(LLState)
  Enable Condition (EnaC)/1(EnaC_stLDWEnaCSyn) -> LLSMCon_stLDWEnaCSyn/1
  Disable Condition (DisblC)/2(DisblC_stLKADisblCSyn) -> LLSMCon_stLKADisblCSyn/1
  Disable Condition (DisblC)/1(DisblC_stLDWDisblCSyn) -> LLSMCon_stLDWDisblCSyn/1
  Enable Condition (EnaC)/2(EnaC_stLKAEnaCSyn) -> LLSMCon_stLKAEnaCSyn/1

== system D53_LKAS_JLU_20200903_0931/LLClb_bsLLClb_Read_Num=100/Subsystem2/Subsystem2/If Action Subsystem ==
  In1 : Inport
  Action Port : ActionPort  ActionType=then
  Out1 : Outport
  wires:
  In1/1 -> Out1/1

== system D53_LKAS_JLU_20200903_0931/LLClb_bsLLClb_Read_Num=100/Subsystem2/Subsystem2/If Action Subsystem1 ==
  In1 : Inport
  Action Port : ActionPort  ActionType=elseif
  Out1 : Outport
  wires:
  In1/1 -> Out1/1

== system D53_LKAS_JLU_20200903_0931/LLClb_bsLLClb_Read_Num=100/Subsystem2/Subsystem2/If Action Subsystem2 ==
  In1 : Inport
  Action Port : ActionPort  ActionType=elseif
  Out1 : Outport
  wires:
  In1/1 -> Out1/1

== system D53_LKAS_JLU_20200903_0931/LLClb_bsLLClb_Read_Num=100/Subsystem2/Subsystem2/If Action Subsystem3 ==
  In1 : Inport
  Action Port : ActionPort  ActionType=elseif
  Out1 : Outport
  wires:
  In1/1 -> Out1/1

== system D53_LKAS_JLU_20200903_0931/LLClb_bsLLClb_Read_Num=100/Subsystem2/Subsystem2/If Action Subsystem4 ==
  In1 : Inport
  Action Port : ActionPort  ActionType=elseif
  Out1 : Outport
  wires:
  In1/1 -> Out1/1

== system D53_LKAS_JLU_20200903_0931/LLClb_bsLLClb_Read_Num=100/Subsystem2/Subsystem2/If Action Subsystem5 ==
  In1 : Inport
  Action Port : ActionPort  ActionType=elseif
  Out1 : Outport
  wires:
  In1/1 -> Out1/1

== system D53_LKAS_JLU_20200903_0931/LLClb_bsLLClb_Read_Num=100/Subsystem2/Subsystem2/If Action Subsystem6 ==
  In1 : Inport
  Action Port : ActionPort  ActionType=elseif
  Out1 : Outport
  wires:
  In1/1 -> Out1/1

== system D53_LKAS_JLU_20200903_0931/LLClb_bsLLClb_Read_Num=100/Subsystem2/Subsystem2/If Action Subsystem7 ==
  In1 : Inport
  Action Port : ActionPort  ActionType=elseif
  Out1 : Outport
  wires:
  In1/1 -> Out1/1

== system D53_LKAS_JLU_20200903_0931/LLClb_bsLLClb_Read_Num=100/Subsystem2/Subsystem2/If Action Subsystem8 ==
  In1 : Inport
  Action Port : ActionPort  ActionType=elseif
  Out1 : Outport
  wires:
  In1/1 -> Out1/1

== system D53_LKAS_JLU_20200903_0931/LLClb_bsLLClb_Read_Num=100/Subsystem2/Subsystem2/If Action Subsystem9 ==
  In1 : Inport
  Action Port : ActionPort  ActionType=elseif
  Out1 : Outport
  wires:
  In1/1 -> Out1/1

== system D53_LKAS_JLU_20200903_0931/LLClb_bsLLClb_Read_Num=100/Subsystem3/Subsystem2/If Action Subsystem ==
  In1 : Inport
  Action Port : ActionPort  ActionType=then
  Out1 : Outport
  wires:
  In1/1 -> Out1/1

== system D53_LKAS_JLU_20200903_0931/LLClb_bsLLClb_Read_Num=100/Subsystem3/Subsystem2/If Action Subsystem1 ==
  In1 : Inport
  Action Port : ActionPort  ActionType=elseif
  Out1 : Outport
  wires:
  In1/1 -> Out1/1

== system D53_LKAS_JLU_20200903_0931/LLClb_bsLLClb_Read_Num=100/Subsystem3/Subsystem2/If Action Subsystem2 ==
  In1 : Inport
  Action Port : ActionPort  ActionType=elseif
  Out1 : Outport
  wires:
  In1/1 -> Out1/1

== system D53_LKAS_JLU_20200903_0931/LLClb_bsLLClb_Read_Num=100/Subsystem3/Subsystem2/If Action Subsystem3 ==
  In1 : Inport
  Action Port : ActionPort  ActionType=elseif
  Out1 : Outport
  wires:
  In1/1 -> Out1/1

== system D53_LKAS_JLU_20200903_0931/LLClb_bsLLClb_Read_Num=100/Subsystem3/Subsystem2/If Action Subsystem4 ==
  In1 : Inport
  Action Port : ActionPort  ActionType=elseif
  Out1 : Outport
  wires:
  In1/1 -> Out1/1

== system D53_LKAS_JLU_20200903_0931/LLClb_bsLLClb_Read_Num=100/Subsystem3/Subsystem2/If Action Subsystem5 ==
  In1 : Inport
  Action Port : ActionPort  ActionType=elseif
  Out1 : Outport
  wires:
  In1/1 -> Out1/1

== system D53_LKAS_JLU_20200903_0931/LLClb_bsLLClb_Read_Num=100/Subsystem3/Subsystem2/If Action Subsystem6 ==
  In1 : Inport
  Action Port : ActionPort  ActionType=elseif
  Out1 : Outport
  wires:
  In1/1 -> Out1/1

== system D53_LKAS_JLU_20200903_0931/LLClb_bsLLClb_Read_Num=100/Subsystem3/Subsystem2/If Action Subsystem7 ==
  In1 : Inport
  Action Port : ActionPort  ActionType=elseif
  Out1 : Outport
  wires:
  In1/1 -> Out1/1

== system D53_LKAS_JLU_20200903_0931/LLClb_bsLLClb_Read_Num=100/Subsystem3/Subsystem2/If Action Subsystem8 ==
  In1 : Inport
  Action Port : ActionPort  ActionType=elseif
  Out1 : Outport
  wires:
  In1/1 -> Out1/1

== system D53_LKAS_JLU_20200903_0931/LLClb_bsLLClb_Read_Num=100/Subsystem3/Subsystem2/If Action Subsystem9 ==
  In1 : Inport
  Action Port : ActionPort  ActionType=elseif
  Out1 : Outport
  wires:
  In1/1 -> Out1/1

== system D53_LKAS_JLU_20200903_0931/LLClb_bsLLClb_Read_Num=100/Subsystem4/Subsystem2/If Action Subsystem ==
  In1 : Inport
  Action Port : ActionPort  ActionType=then
  Out1 : Outport
  wires:
  In1/1 -> Out1/1

== system D53_LKAS_JLU_20200903_0931/LLClb_bsLLClb_Read_Num=100/Subsystem4/Subsystem2/If Action Subsystem1 ==
  In1 : Inport
  Action Port : ActionPort  ActionType=elseif
  Out1 : Outport
  wires:
  In1/1 -> Out1/1

== system D53_LKAS_JLU_20200903_0931/LLClb_bsLLClb_Read_Num=100/Subsystem4/Subsystem2/If Action Subsystem2 ==
  In1 : Inport
  Action Port : ActionPort  ActionType=elseif
  Out1 : Outport
  wires:
  In1/1 -> Out1/1

== system D53_LKAS_JLU_20200903_0931/LLClb_bsLLClb_Read_Num=100/Subsystem4/Subsystem2/If Action Subsystem3 ==
  In1 : Inport
  Action Port : ActionPort  ActionType=elseif
  Out1 : Outport
  wires:
  In1/1 -> Out1/1

== system D53_LKAS_JLU_20200903_0931/LLClb_bsLLClb_Read_Num=100/Subsystem4/Subsystem2/If Action Subsystem4 ==
  In1 : Inport
  Action Port : ActionPort  ActionType=elseif
  Out1 : Outport
  wires:
  In1/1 -> Out1/1

== system D53_LKAS_JLU_20200903_0931/LLClb_bsLLClb_Read_Num=100/Subsystem4/Subsystem2/If Action Subsystem5 ==
  In1 : Inport
  Action Port : ActionPort  ActionType=elseif
  Out1 : Outport
  wires:
  In1/1 -> Out1/1

== system D53_LKAS_JLU_20200903_0931/LLClb_bsLLClb_Read_Num=100/Subsystem4/Subsystem2/If Action Subsystem6 ==
  In1 : Inport
  Action Port : ActionPort  ActionType=elseif
  Out1 : Outport
  wires:
  In1/1 -> Out1/1

== system D53_LKAS_JLU_20200903_0931/LLClb_bsLLClb_Read_Num=100/Subsystem4/Subsystem2/If Action Subsystem7 ==
  In1 : Inport
  Action Port : ActionPort  ActionType=elseif
  Out1 : Outport
  wires:
  In1/1 -> Out1/1

== system D53_LKAS_JLU_20200903_0931/LLClb_bsLLClb_Read_Num=100/Subsystem4/Subsystem2/If Action Subsystem8 ==
  In1 : Inport
  Action Port : ActionPort  ActionType=elseif
  Out1 : Outport
  wires:
  In1/1 -> Out1/1

== system D53_LKAS_JLU_20200903_0931/LLClb_bsLLClb_Read_Num=100/Subsystem4/Subsystem2/If Action Subsystem9 ==
  In1 : Inport
  Action Port : ActionPort  ActionType=elseif
  Out1 : Outport
  wires:
  In1/1 -> Out1/1

== system D53_LKAS_JLU_20200903_0931/LL/LL Inputs Mapping/bsLaneInfo/LaneSelect/Subsystem ==
  R0_Q_In : Inport
  Constant1 : Constant  Value=3  OutDataTypeStr=uint8
  Switch1 : Switch  Threshold=2
  R0_Q : Outport
  wires:
  Constant1/1 -> Switch1/1
  R0_Q_In/1 -> Switch1/2, Switch1/3
  Switch1/1 -> R0_Q/1  "R0_Q"

== system D53_LKAS_JLU_20200903_0931/LL/LL Inputs Mapping/bsLaneInfo/LaneSelect/Subsystem1 ==
  R0_Q_In : Inport
  Constant1 : Constant  Value=3  OutDataTypeStr=uint8
  Switch1 : Switch  Threshold=2
  R0_Q : Outport
  wires:
  Switch1/1 -> R0_Q/1  "R0_Q"
  R0_Q_In/1 -> Switch1/3, Switch1/2
  Constant1/1 -> Switch1/1

== system D53_LKAS_JLU_20200903_0931/LL/LL Inputs Mapping/bsLaneInfo/LaneSelect/Subsystem2 ==
  L0_Q_In : Inport
  Constant : Constant  Value=3  OutDataTypeStr=uint8
  Switch : Switch  Threshold=2
  L0_Q : Outport
  wires:
  Switch/1 -> L0_Q/1  "L0_Q"
  Constant/1 -> Switch/1
  L0_Q_In/1 -> Switch/2, Switch/3

== system D53_LKAS_JLU_20200903_0931/LL/LL Inputs Mapping/bsLaneInfo/LaneSelect/Subsystem4 ==
  L0_Q_In : Inport
  Constant : Constant  Value=3  OutDataTypeStr=uint8
  Switch : Switch  Threshold=2
  L0_Q : Outport
  wires:
  L0_Q_In/1 -> Switch/3, Switch/2
  Constant/1 -> Switch/1
  Switch/1 -> L0_Q/1  "L0_Q"

== system D53_LKAS_JLU_20200903_0931/LL/LL Inputs Mapping/bsLaneInfo/LanesReconstruct /Left 1Lane Reconstruct (Lft1LaneR) ==
  stFlag : Inport
  bsL1Info : Inport  Port=2
  Bus Creator2 : BusCreator  Inputs=10
  Bus Selector1 : BusSelector  OutputSignals=L1_C0,L1_C1,L1_C2,L1_C3,L1_VR,L1_Q,L1_Type,L1_W,L1_TLC,L1_LC
  Constant : Constant  Value=0  OutDataTypeStr=uint16
  Switch3 : Switch  Criteria=u2 > Threshold
  bsL1InfoR : Outport
  wires:
  Bus Selector1/1 -> Bus Creator2/1  "<L1_C0>"
  Bus Selector1/2 -> Bus Creator2/2  "<L1_C1>"
  Bus Selector1/3 -> Bus Creator2/3  "<L1_C2>"
  Bus Selector1/4 -> Bus Creator2/4  "<L1_C3>"
  Bus Creator2/1 -> bsL1InfoR/1  "bsL1Info"
  Switch3/1 -> Bus Creator2/6  "L1_Q"
  Constant/1 -> Switch3/3
  Bus Selector1/6 -> Switch3/1  "<L1_Q>"
  stFlag/1 -> Switch3/2
  bsL1Info/1 -> Bus Selector1/1
  Bus Selector1/5 -> Bus Creator2/5  "<L1_VR>"
  Bus Selector1/7 -> Bus Creator2/7  "<L1_Type>"
  Bus Selector1/8 -> Bus Creator2/8  "<L1_W>"
  Bus Selector1/10 -> Bus Creator2/10  "<L1_LC>"
  Bus Selector1/9 -> Bus Creator2/9  "<L1_TLC>"
